simulink model "SB9_continuous_done"  (R2024b)
settings: Solver=ode45  StartTime=0.0  StopTime=5  MaxStep=0.01  RelTol=1e-3
settings Model: Creator=admin  LastModifiedBy=admin

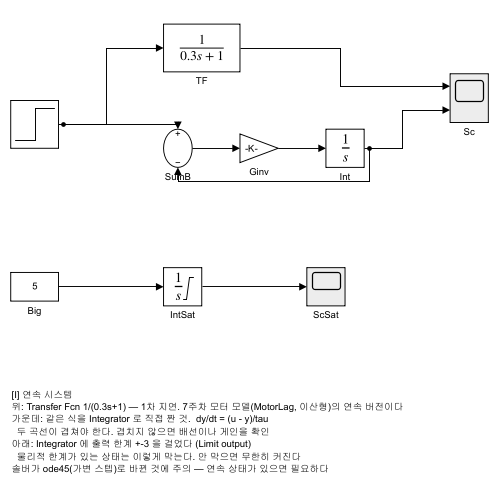
[thumbnail: Simulink's stored preview of the top-level diagram]
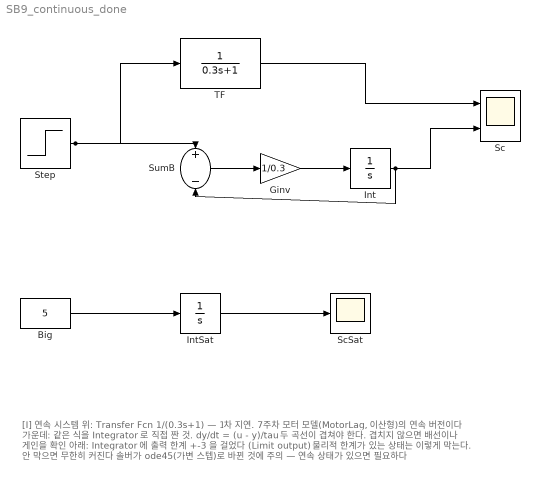
== system SB9_continuous_done ==
  note: [I] 연속 시스템
      | 위: Transfer Fcn 1/(0.3s+1) — 1차 지연. 7주차 모터 모델(MotorLag, 이산형)의 연속 버전이다
      | 가운데: 같은 식을 Integrator 로 직접 짠 것.  dy/dt = (u - y)/tau
      |   두 곡선이 겹쳐야 한다. 겹치지 않으면 배선이나 게인을 확인
      | 아래: Integrator 에 출력 한계 +-3 을 걸었다 (Limit output)
      |   물리적 한계가 있는 상태는 이렇게 막는다. 안 막으면 무한히 커진다
      | 솔버가 ode45(가변 스텝)로 바뀐 것에 주의 — 연속 상태가 있으면 필요하다
  Big : Constant  Value=5
  Ginv : Gain  Gain=1/0.3
  Int : Integrator
  IntSat : Integrator  LimitOutput=on  UpperSaturationLimit=3  LowerSaturationLimit=-3
  Sc : Scope  NumInputPorts=2
  ScSat : Scope
  Step : Step  SampleTime=0
  SumB : Sum  Inputs=+-
  TF : TransferFcn  Denominator=[0.3 1]
  wires:
  Step/1 -> TF/1, SumB/1
  TF/1 -> Sc/1
  SumB/1 -> Ginv/1
  Ginv/1 -> Int/1
  Int/1 -> SumB/2, Sc/2
  Big/1 -> IntSat/1
  IntSat/1 -> ScSat/1
